simulink model "ELECTRIC_RC_AIRCRAFT_simulink_backup_3"  (R2025b)
settings: Solver=VariableStepAuto  StartTime=0.0  StopTime=1000  RelTol=1e-3
values from neighbouring files (symbols this model uses):
  AoA = [-5 0 5 10 15]    [ELECTRIC_RC_AIRCRAFT.m]
  C_mq = -2*((Tail_Wing_Area/Wing_Surface_Area)*(tail_moment_arm/chord_length_tail))    (= -0.900546448087)    [ELECTRIC_RC_AIRCRAFT.m]
  C_mse = -n*(Tail_Wing_Area/Wing_Surface_Area)*(tail_moment_arm/chord_length_tail)    (= -0.351213114754)    [ELECTRIC_RC_AIRCRAFT.m]
  chord_length = 0.25    [ELECTRIC_RC_AIRCRAFT.m]
  CL = [-0.249 0.205 0.752 1.190 1.316]    [ELECTRIC_RC_AIRCRAFT.m]
  CM = [0.0550 0.0260 -0.0854 -0.1805]    [ELECTRIC_RC_AIRCRAFT.m]
  g = 9.81    [ELECTRIC_RC_AIRCRAFT.m]
  Inertia = (m/12)*(fuselage_length^2+wing_span^2)    (= 0.54883225)    [ELECTRIC_RC_AIRCRAFT.m]
  m = 1.83    [ELECTRIC_RC_AIRCRAFT.m]
  Velocity_initial = 20    [ELECTRIC_RC_AIRCRAFT.m]
  Wing_Surface_Area = 0.4575    [ELECTRIC_RC_AIRCRAFT.m]
libraries: aerolibconvert2 x4, slpidlib x3, aerolibadyn x1, aerolibasang x1, aerolibbdyn x1, aerolibactuator x1, simulink x1, aerolibpropulsion2 x1
settings Model: Creator=papar  LastModifiedBy=papar

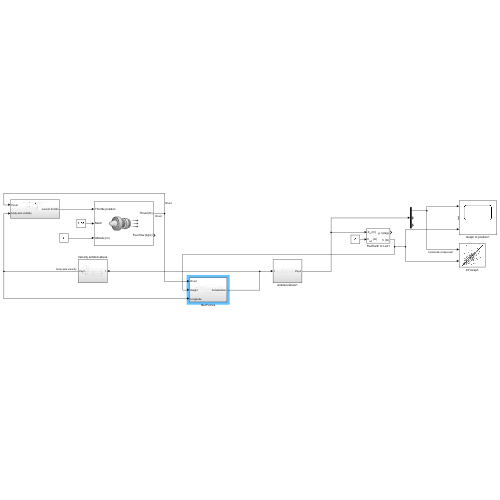
[thumbnail: Simulink's stored preview of the top-level diagram]
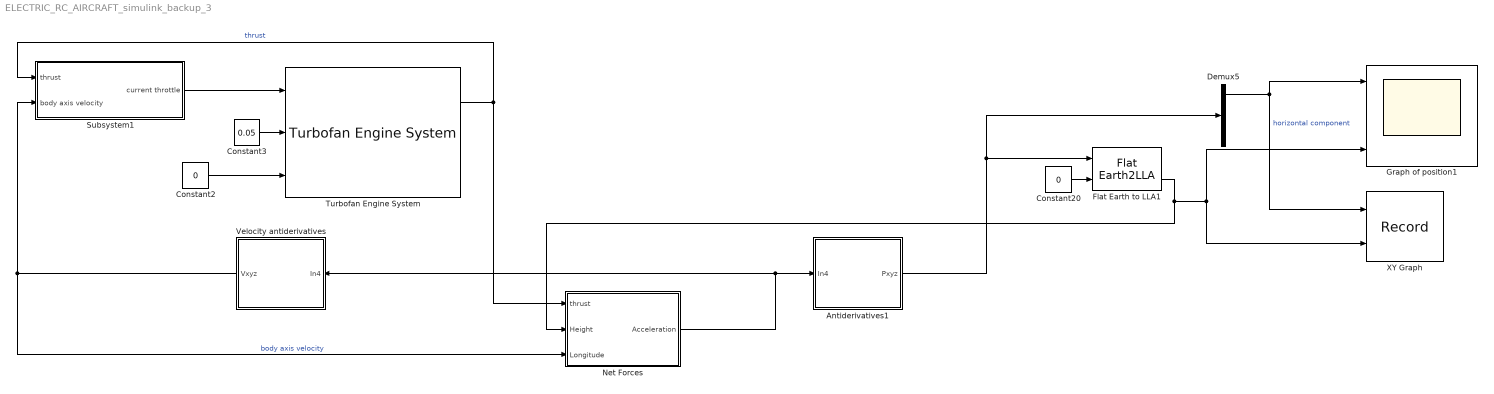
== system ELECTRIC_RC_AIRCRAFT_simulink_backup_3 ==
  Antiderivatives1 : Subsystem
  Constant2 : Constant  Value=0
  Constant20 : Constant  Value=0
  Constant3 : Constant  Value=0.05
  Demux5 : Demux  Outputs=3
  Flat Earth to LLA1 : FlatEarth2LLA
  Graph of position1 : Scope  NumInputPorts=3
      settings: ActiveDisplayYMinimum=-1.9016190813754986E+6  ActiveDisplayYMaximum=1.43321045610095E+6
  Net Forces : Subsystem
  Subsystem1 : Subsystem
  Turbofan Engine System : aerolibpropulsion2/Turbofan Engine System  units=Metric (MKS)  ic_source=Internal  IC=50  Fmax=50  tau=0.4  SFC=0  Nt=0.9
  Velocity antiderivatives : Subsystem
  XY Graph : Record  NumPorts=2.0  FileSettingsInternal="{\"entries\":[{\"content\":{\"excelSettings\":{\"content\":{},\"type\":\"Streamout.ExcelSettings\"},\"parquetSettings\":{\"content\":{},\"type\":\"Streamout.ParquetSettings\"}},\"type\":\"Streamout.FileSettingStorage\",\"uuid\":\"\"}],\"packageUris\":[\"http:\\/\\/schema.mathworks.com\\/mf0\\/streamout_blocks\\/R2020a\"],\"version\":\"1.0\"}"  FrameSettings=[0, 0]  Layout=[1 1]  SignalsInternal="{\"entries\":[{\"content\":{\"signals\":[{\"content\":{\"blockPath\":[],\"dimensions\":[1],\"domain\":\"\",\"lineColor\":\"#a2142f\",\"plots\":[ 1 ],\"port\":1,\"sid\":[\"\"],\"signalID\":1,\"signalName\":\"horizontal component\"},\"type\":\"RecordBlkView.Signal\",\"uuid\":\"\"},{\"content\":{\"blockPath\":[],\"dimensions\":[1],\"domain\":\"\",\"lineColor\":\"#139fff\",\"plots\":[ 1 ],\"port\":2,\"sid\":[\"\"],\"signalID\":2,\"signalName\":\"Flat Earth to LLA1:2\"},\"type\":\"RecordBlkView.Signal\",\"uuid\":\"\"}]},\"type\":\"RecordBlkView.InputSignals\",\"uuid\":\"\"}],\"packageUris\":[\"http:\\/\\/schema.mathworks.com\\/mf0\\/streamout_blocks\\/R2020a\"],\"version\":\"1.0\"}"  VisualizationBindings="{\"xyplotplugin\":{\"info\":[{\"series\":[{\"bindingParametersList\":[{\"parameter\":\"X-Axis\",\"signalID\":1,\"signalName\":\"horizontal component\"},{\"parameter\":\"Y-Axis\",\"signalID\":2,\"signalName\":\"Flat Earth to LLA1:2\"}],\"seriesID\":0}],\"subplotID\":1}]}}"  CompatibilityTag=XY
  wires:
  Constant2/1 -> Turbofan Engine System/3
  Constant3/1 -> Turbofan Engine System/2
  Antiderivatives1/1(Pxyz) -> Demux5/1, Flat Earth to LLA1/1
  Constant20/1 -> Flat Earth to LLA1/2
  Demux5/1 -> Graph of position1/1, XY Graph/1  "horizontal component"
  Flat Earth to LLA1/2 -> Net Forces/2(Height), Graph of position1/3, XY Graph/2
  Velocity antiderivatives/1(Vxyz) -> Net Forces/3(Longitude), Subsystem1/2(body axis velocity)  "body axis velocity"
  Net Forces/1(Acceleration) -> Antiderivatives1/1(In4), Velocity antiderivatives/1(In4)
  Turbofan Engine System/1 -> Subsystem1/1(thrust), Net Forces/1(thrust)  "thrust"
  Subsystem1/1(current throttle) -> Turbofan Engine System/1

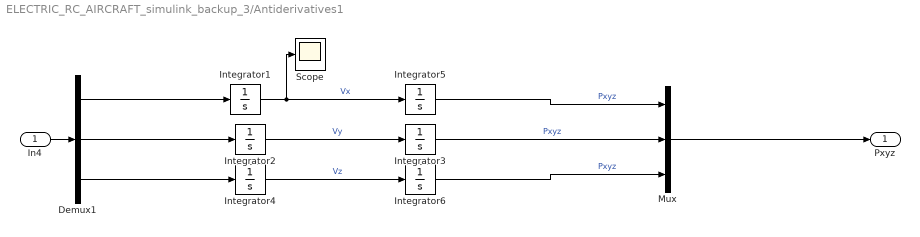
== system ELECTRIC_RC_AIRCRAFT_simulink_backup_3/Antiderivatives1 ==
  In4 : Inport
  Demux1 : Demux  Outputs=3
  Integrator1 : Integrator  InitialCondition=Velocity_initial  UpperSaturationLimit=30  LowerSaturationLimit=-10
  Integrator{2..6} (5 alike) : Integrator
  Mux : Mux  Inputs=3
  Scope : Scope
      settings: ActiveDisplayYMinimum=-71.95223956202382  ActiveDisplayYMaximum=46.668491481612783  DataLoggingVariableName=ScopeData4
  Pxyz : Outport
  wires:
  Integrator2/1 -> Integrator3/1  "Vy"
  In4/1 -> Demux1/1
  Integrator1/1 -> Scope/1, Integrator5/1  "Vx"
  Demux1/2 -> Integrator2/1
  Demux1/1 -> Integrator1/1
  Demux1/3 -> Integrator4/1
  Integrator4/1 -> Integrator6/1  "Vz"
  Mux/1 -> Pxyz/1
  Integrator3/1 -> Mux/2  "Pxyz"
  Integrator5/1 -> Mux/1  "Pxyz"
  Integrator6/1 -> Mux/3  "Pxyz"

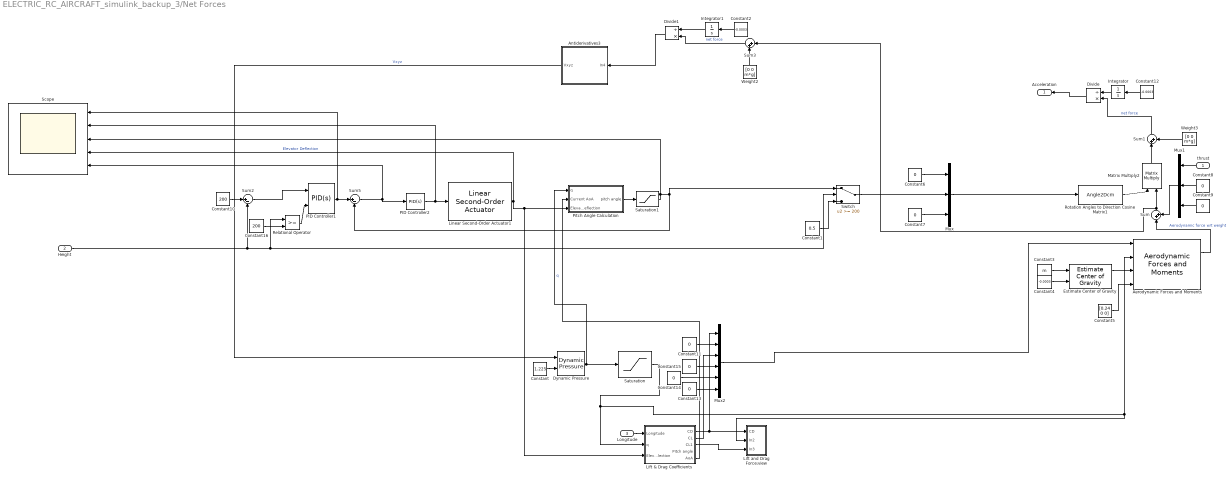
== system ELECTRIC_RC_AIRCRAFT_simulink_backup_3/Net Forces ==
  thrust : Inport
  Height : Inport  Port=2
  Longitude : Inport  Port=3
  "Aerodynamic Forces and Moments " : aerolibadyn/Aerodynamic Forces and Moments   inputAxes=Body  outputForceAxes=Body  outputMomentAxes=Body  S=Wing_Surface_Area  b=1.83  cbar=0.25
  Antiderivatives3 : Subsystem
  Constant : Constant  Value=1.225
  Constant1 : Constant  Value=0.5
  Constant10 : Constant  Value=200
  Constant{6..9,11,13..15} (8 alike) : Constant  Value=0
  Constant12 : Constant  Value=-0.0003
  Constant16 : Constant  Value=200
  Constant2 : Constant  Value=-0.0003
  Constant3 : Constant  Value=m
  Constant4 : Constant  Value=-0.0003
  Constant5 : Constant  Value=[0.24 0 0]
  Divide : Product  Inputs=/*
  Divide1 : Product  Inputs=/*
  Dynamic Pressure : aerolibasang/Dynamic Pressure
  Estimate Center of Gravity : aerolibbdyn/Estimate Center of Gravity  fmass=m  emass=1.63  fcg=[0.24 0 0]'  ecg=[0.23 0 0]'
  Integrator : Integrator  InitialCondition=m  LimitOutput=on  UpperSaturationLimit=1.83  LowerSaturationLimit=1.53
  Integrator1 : Integrator  InitialCondition=m  LimitOutput=on  UpperSaturationLimit=1.83  LowerSaturationLimit=1.53
  Lift & Drag Coefficients : Subsystem
  Lift and Drag Force:view : Subsystem
  Linear Second-Order Actuator1 : aerolibactuator/Linear Second-Order Actuator  wn_fin=8  z_fin=0.7  fin_act_0=0  fin_act_vel=0
  Matrix Multiply2 : Product  Multiplication=Matrix(*)
  Mux : Mux  Inputs=3
  Mux1 : Mux  Inputs=3
  Mux2 : Mux  Inputs=6
  PID Controller1 : slpidlib/PID Controller  Controller=PID  Form=Parallel  TimeDomain=Continuous-time  UseExternalTs=off  SampleTime=-1  IntegratorMethod=Forward Euler  FilterMethod=Forward Euler  ControllerParametersSource=internal  P=1.0E-2  I=0  UseKiTs=off  D=0  UseExternalDerivativeSource=off  N=10  UseFilter=on  TunerSelectOption=Transfer Function Based (PID Tuner App)  InitialConditionSource=internal  InitialConditionForIntegrator=0  InitialConditionForFilter=0  DifferentiatorICPrevScaledInput=0  ExternalReset=rising  TrackingMode=off  Kt=1  LimitOutput=on  SatLimitsSource=internal  UpperSaturationLimit=0.087  LowerSaturationLimit=-0.087  LinearizeAsGain=on  AntiWindupMode=none  Kb=1  LimitIntegrator=off  UpperIntegratorSaturationLimit=inf  LowerIntegratorSaturationLimit=-inf  POutMin=[]  POutMax=[]  IOutMin=[]  IOutMax=[]  DOutMin=[]  DOutMax=[]  NOutMin=[]  NOutMax=[]  SumOutMin=[]  SumOutMax=[]  SaturationOutMin=[]  SaturationOutMax=[]  PParamMin=[]  PParamMax=[]  IParamMin=[]  IParamMax=[]  DParamMin=[]  DParamMax=[]  NParamMin=[]  NParamMax=[]  KbParamMin=[]  KbParamMax=[]  KtParamMin=[]  KtParamMax=[]  KbOutMin=[]  KbOutMax=[]  KtOutMin=[]  KtOutMax=[]  IntegratorOutMin=[]  IntegratorOutMax=[]  FilterOutMin=[]  FilterOutMax=[]  SumI1OutMin=[]  SumI1OutMax=[]  SumI2OutMin=[]  SumI2OutMax=[]  SumI3OutMin=[]  SumI3OutMax=[]  SumI4OutMin=[]  SumI4OutMax=[]  SumDOutMin=[]  SumDOutMax=[]  DifferentiatorOutMin=[]  DifferentiatorOutMax=[]  FilterDiffOutCoefMin=[]  FilterDiffOutCoefMax=[]  ReciprocalOutMin=[]  ReciprocalOutMax=[]  SumDenOutMin=[]  SumDenOutMax=[]  SumNumOutMin=[]  SumNumOutMax=[]  DivideOutMin=[]  DivideOutMax=[]  UdiffTsProdOutMin=[]  UdiffTsProdOutMax=[]  NTsProdOutMin=[]  NTsProdOutMax=[]  UintegralTsProdOutMin=[]  UintegralTsProdOutMax=[]  UngainTsProdOutMin=[]  UngainTsProdOutMax=[]  ClampingZeroOutDataTypeStr=Inherit: Inherit via back propagation  ClampingZeroOutMin=[]  ClampingZeroOutMax=[]  FilterDenConstantOutDataTypeStr=Inherit: Inherit via back propagation  FilterDenConstantOutMin=[]  FilterDenConstantOutMax=[]  PCopyOutDataTypeStr=Inherit: Inherit via back propagation  PCopyOutMin=[]  PCopyOutMax=[]  NCopyOutDataTypeStr=Inherit: Inherit via back propagation  NCopyOutMin=[]  NCopyOutMax=[]  IntegratorContinuousStateAttributes=''  IntegratorStateMustResolveToSignalObject=off  IntegratorRTWStateStorageClass=Auto  FilterContinuousStateAttributes=''  FilterStateMustResolveToSignalObject=off  FilterRTWStateStorageClass=Auto  ParallelPVariant=InternalParameters  IdealPVariant=Disabled  IVariant=InternalParameters  DVariant=InternalParameters  IntegratorVariant=Continuous  SatVariant=Enabled  AWVariant=Passthrough  PCopyVariant=Disabled  TRVariant=Disabled  FdbkBlocksVariant=Forward  IdealPFdbkVariant=Disabled  SatFdbkVariant=Disabled  DerivativeFilterVariant=ContFilter  NVariant=InternalParameters  NCopyVariant=Disabled  FilterICVariant=InternalICsFilter  IntegratorICVariant=InternalICs  ExternalResetVariant=ExternalReset  TRSumVariant=Passthrough  SumFdbkVariant=Disabled  SumVariant=Sum_PID  TsampFilterVariant=InternalTs  TsampNgainVariant=Passthrough  TsampIntegralVariant=Disabled_SignalSpec  ExternalSaturationOutDataTypeStr=Inherit: Same as second input  DerivativeSourceVariant=ErrorSignal  PreIntVariant=InternalPreInt
  PID Controller2 : slpidlib/PID Controller  Controller=PID  Form=Parallel  TimeDomain=Continuous-time  UseExternalTs=off  SampleTime=-1  IntegratorMethod=Forward Euler  FilterMethod=Forward Euler  ControllerParametersSource=internal  P=1.0E-3  I=0  UseKiTs=off  D=1.0E-3  UseExternalDerivativeSource=off  N=20  UseFilter=on  TunerSelectOption=Transfer Function Based (PID Tuner App)  InitialConditionSource=internal  InitialConditionForIntegrator=0  InitialConditionForFilter=0  DifferentiatorICPrevScaledInput=0  ExternalReset=none  TrackingMode=off  Kt=1  LimitOutput=off  SatLimitsSource=internal  UpperSaturationLimit=inf  LowerSaturationLimit=-inf  LinearizeAsGain=on  AntiWindupMode=none  Kb=1  LimitIntegrator=off  UpperIntegratorSaturationLimit=inf  LowerIntegratorSaturationLimit=-inf  POutMin=[]  POutMax=[]  IOutMin=[]  IOutMax=[]  DOutMin=[]  DOutMax=[]  NOutMin=[]  NOutMax=[]  SumOutMin=[]  SumOutMax=[]  SaturationOutMin=[]  SaturationOutMax=[]  PParamMin=[]  PParamMax=[]  IParamMin=[]  IParamMax=[]  DParamMin=[]  DParamMax=[]  NParamMin=[]  NParamMax=[]  KbParamMin=[]  KbParamMax=[]  KtParamMin=[]  KtParamMax=[]  KbOutMin=[]  KbOutMax=[]  KtOutMin=[]  KtOutMax=[]  IntegratorOutMin=[]  IntegratorOutMax=[]  FilterOutMin=[]  FilterOutMax=[]  SumI1OutMin=[]  SumI1OutMax=[]  SumI2OutMin=[]  SumI2OutMax=[]  SumI3OutMin=[]  SumI3OutMax=[]  SumI4OutMin=[]  SumI4OutMax=[]  SumDOutMin=[]  SumDOutMax=[]  DifferentiatorOutMin=[]  DifferentiatorOutMax=[]  FilterDiffOutCoefMin=[]  FilterDiffOutCoefMax=[]  ReciprocalOutMin=[]  ReciprocalOutMax=[]  SumDenOutMin=[]  SumDenOutMax=[]  SumNumOutMin=[]  SumNumOutMax=[]  DivideOutMin=[]  DivideOutMax=[]  UdiffTsProdOutMin=[]  UdiffTsProdOutMax=[]  NTsProdOutMin=[]  NTsProdOutMax=[]  UintegralTsProdOutMin=[]  UintegralTsProdOutMax=[]  UngainTsProdOutMin=[]  UngainTsProdOutMax=[]  ClampingZeroOutDataTypeStr=Inherit: Inherit via back propagation  ClampingZeroOutMin=[]  ClampingZeroOutMax=[]  FilterDenConstantOutDataTypeStr=Inherit: Inherit via back propagation  FilterDenConstantOutMin=[]  FilterDenConstantOutMax=[]  PCopyOutDataTypeStr=Inherit: Inherit via back propagation  PCopyOutMin=[]  PCopyOutMax=[]  NCopyOutDataTypeStr=Inherit: Inherit via back propagation  NCopyOutMin=[]  NCopyOutMax=[]  IntegratorContinuousStateAttributes=''  IntegratorStateMustResolveToSignalObject=off  IntegratorRTWStateStorageClass=Auto  FilterContinuousStateAttributes=''  FilterStateMustResolveToSignalObject=off  FilterRTWStateStorageClass=Auto  ParallelPVariant=InternalParameters  IdealPVariant=Disabled  IVariant=InternalParameters  DVariant=InternalParameters  IntegratorVariant=Continuous  SatVariant=Disabled  AWVariant=Passthrough  PCopyVariant=Disabled  TRVariant=Disabled  FdbkBlocksVariant=Forward  IdealPFdbkVariant=Disabled  SatFdbkVariant=Disabled  DerivativeFilterVariant=ContFilter  NVariant=InternalParameters  NCopyVariant=Disabled  FilterICVariant=InternalICsFilter  IntegratorICVariant=InternalICs  ExternalResetVariant=Disabled  TRSumVariant=Passthrough  SumFdbkVariant=Disabled  SumVariant=Sum_PID  TsampFilterVariant=InternalTs  TsampNgainVariant=Passthrough  TsampIntegralVariant=Disabled_SignalSpec  ExternalSaturationOutDataTypeStr=Inherit: Same as second input  DerivativeSourceVariant=ErrorSignal  PreIntVariant=InternalPreInt
  Pitch Angle Calculation : Subsystem
  Relational Operator : RelationalOperator  OutDataTypeStr=boolean  RndMeth=Simplest  InputSameDT=off
  Rotation Angles to Direction Cosine Matrix1 : Angle2Dcm  rotationOrder=XYZ
      settings: AttributesFormatString=Rotation Order: %<rotationOrder>
  Saturation : Saturate  UpperLimit=200  LowerLimit=0
  Saturation1 : Saturate  UpperLimit=0.1  LowerLimit=-1.7
  Scope : Scope  NumInputPorts=5
      settings: ActiveDisplayYMinimum=-6.4413632870801404E+7  ActiveDisplayYMaximum=4.62135418449443E+7  DataLoggingVariableName=ScopeData2
  Sum : Sum  Inputs=|++
  Sum1 : Sum  Inputs=|++
  Sum2 : Sum  Inputs=|+-
  Sum3 : Sum  Inputs=|++
  Sum5 : Sum  Inputs=|+-
  Switch : Switch  Threshold=200  SaturateOnIntegerOverflow=off  InputSameDT=off
  Weight2 : Constant  Value=[0 0 m*g]
  Weight3 : Constant  Value=[0 0 m*g]
  Acceleration : Outport
  wires:
  Constant5/1 -> "Aerodynamic Forces and Moments "/4
  Saturation/1 -> Lift & Drag Coefficients/2(q), "Aerodynamic Forces and Moments "/2, Lift and Drag Force:view/2(In2)
  Lift & Drag Coefficients/1(CD) -> Mux2/1, Lift and Drag Force:view/1(CD)
  Longitude/1 -> Lift & Drag Coefficients/1(Longitude)
  Constant8/1 -> Mux1/2
  Constant/1 -> Dynamic Pressure/2
  Dynamic Pressure/1 -> Saturation/1, Pitch Angle Calculation/1(q)  "q"
  Rotation Angles to Direction Cosine Matrix1/1 -> Matrix Multiply2/1
  Mux1/1 -> Sum/2
  Constant10/1 -> Sum2/1
  Sum/1 -> Matrix Multiply2/2, Sum3/1
  Mux2/1 -> "Aerodynamic Forces and Moments "/1
  thrust/1 -> Mux1/1
  Constant11/1 -> Mux2/2
  Estimate Center of Gravity/1 -> "Aerodynamic Forces and Moments "/3
  Weight3/1 -> Sum1/2
  Constant14/1 -> Mux2/5
  Weight2/1 -> Sum3/2
  Antiderivatives3/1(Vxyz) -> Dynamic Pressure/1  "Vxyz"
  Constant6/1 -> Mux/1
  Lift & Drag Coefficients/3(CL1) -> Lift and Drag Force:view/3(In3)
  "Aerodynamic Forces and Moments "/1 -> Sum/1  "Aerodynamic force w/t weight"
  Constant7/1 -> Mux/3
  Matrix Multiply2/1 -> Sum1/1
  Constant9/1 -> Mux1/3
  Constant13/1 -> Mux2/6
  Constant15/1 -> Mux2/4
  Lift & Drag Coefficients/2(CL) -> Mux2/3
  Constant3/1 -> Estimate Center of Gravity/1
  Constant4/1 -> Estimate Center of Gravity/2
  Constant12/1 -> Integrator/1
  Integrator/1 -> Divide/1
  Divide/1 -> Acceleration/1
  Sum1/1 -> Divide/2  "net force"
  Sum3/1 -> Divide1/2  "net force"
  Integrator1/1 -> Divide1/1
  Constant2/1 -> Integrator1/1
  Divide1/1 -> Antiderivatives3/1(In4)
  PID Controller1/1 -> Scope/1, Sum5/1
  Sum5/1 -> PID Controller2/1, Scope/5
  Lift & Drag Coefficients/5(AoA) -> Pitch Angle Calculation/2(Current AoA)
  Pitch Angle Calculation/1(pitch angle) -> Saturation1/1
  Mux/1 -> Rotation Angles to Direction Cosine Matrix1/1
  PID Controller2/1 -> Scope/2, Linear Second-Order Actuator1/1
  Linear Second-Order Actuator1/1 -> Scope/4, Lift & Drag Coefficients/3(Elevator Deflection), Pitch Angle Calculation/3(Elevator Deflection)  "Elevator Deflection"
  Sum2/1 -> PID Controller1/1
  Switch/1 -> Mux/2
  Constant1/1 -> Switch/3
  Height/1 -> Relational Operator/1, Switch/2, Sum2/2
  Saturation1/1 -> Switch/1, Sum5/2, Scope/3
  Constant16/1 -> Relational Operator/2
  Relational Operator/1 -> PID Controller1/2

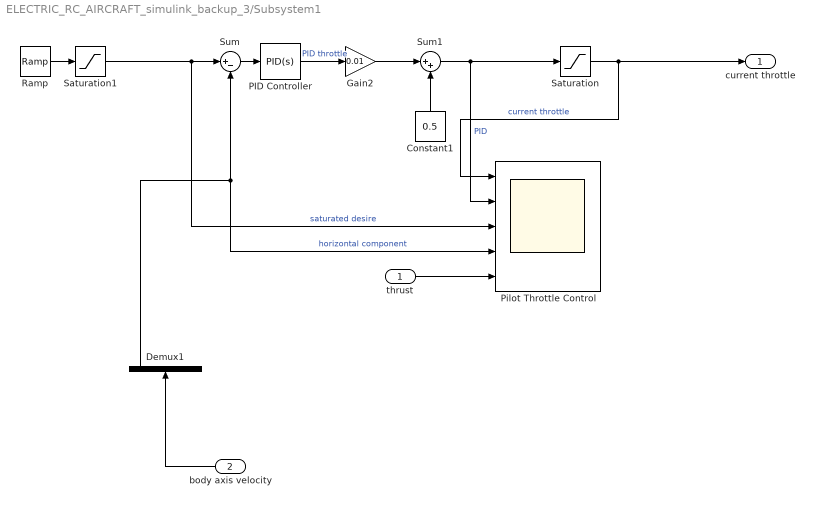
== system ELECTRIC_RC_AIRCRAFT_simulink_backup_3/Subsystem1 ==
  thrust : Inport
  body axis velocity : Inport  Port=2
  Constant1 : Constant  Value=0.5
  Demux1 : Demux  Outputs=3
  Gain2 : Gain  Gain=0.01
  PID Controller : slpidlib/PID Controller  Controller=PID  Form=Parallel  TimeDomain=Continuous-time  UseExternalTs=off  SampleTime=-1  IntegratorMethod=Forward Euler  FilterMethod=Forward Euler  ControllerParametersSource=internal  P=0.5  I=5.0E-3  UseKiTs=off  D=0.1  UseExternalDerivativeSource=off  N=20  UseFilter=on  TunerSelectOption=Transfer Function Based (PID Tuner App)  InitialConditionSource=internal  InitialConditionForIntegrator=0  InitialConditionForFilter=0  DifferentiatorICPrevScaledInput=0  ExternalReset=none  TrackingMode=off  Kt=1  LimitOutput=off  SatLimitsSource=internal  UpperSaturationLimit=inf  LowerSaturationLimit=-inf  LinearizeAsGain=on  AntiWindupMode=none  Kb=1  LimitIntegrator=off  UpperIntegratorSaturationLimit=inf  LowerIntegratorSaturationLimit=-inf  POutMin=[]  POutMax=[]  IOutMin=[]  IOutMax=[]  DOutMin=[]  DOutMax=[]  NOutMin=[]  NOutMax=[]  SumOutMin=[]  SumOutMax=[]  SaturationOutMin=[]  SaturationOutMax=[]  PParamMin=[]  PParamMax=[]  IParamMin=[]  IParamMax=[]  DParamMin=[]  DParamMax=[]  NParamMin=[]  NParamMax=[]  KbParamMin=[]  KbParamMax=[]  KtParamMin=[]  KtParamMax=[]  KbOutMin=[]  KbOutMax=[]  KtOutMin=[]  KtOutMax=[]  IntegratorOutMin=[]  IntegratorOutMax=[]  FilterOutMin=[]  FilterOutMax=[]  SumI1OutMin=[]  SumI1OutMax=[]  SumI2OutMin=[]  SumI2OutMax=[]  SumI3OutMin=[]  SumI3OutMax=[]  SumI4OutMin=[]  SumI4OutMax=[]  SumDOutMin=[]  SumDOutMax=[]  DifferentiatorOutMin=[]  DifferentiatorOutMax=[]  FilterDiffOutCoefMin=[]  FilterDiffOutCoefMax=[]  ReciprocalOutMin=[]  ReciprocalOutMax=[]  SumDenOutMin=[]  SumDenOutMax=[]  SumNumOutMin=[]  SumNumOutMax=[]  DivideOutMin=[]  DivideOutMax=[]  UdiffTsProdOutMin=[]  UdiffTsProdOutMax=[]  NTsProdOutMin=[]  NTsProdOutMax=[]  UintegralTsProdOutMin=[]  UintegralTsProdOutMax=[]  UngainTsProdOutMin=[]  UngainTsProdOutMax=[]  ClampingZeroOutDataTypeStr=Inherit: Inherit via back propagation  ClampingZeroOutMin=[]  ClampingZeroOutMax=[]  FilterDenConstantOutDataTypeStr=Inherit: Inherit via back propagation  FilterDenConstantOutMin=[]  FilterDenConstantOutMax=[]  PCopyOutDataTypeStr=Inherit: Inherit via back propagation  PCopyOutMin=[]  PCopyOutMax=[]  NCopyOutDataTypeStr=Inherit: Inherit via back propagation  NCopyOutMin=[]  NCopyOutMax=[]  IntegratorContinuousStateAttributes=''  IntegratorStateMustResolveToSignalObject=off  IntegratorRTWStateStorageClass=Auto  FilterContinuousStateAttributes=''  FilterStateMustResolveToSignalObject=off  FilterRTWStateStorageClass=Auto  ParallelPVariant=InternalParameters  IdealPVariant=Disabled  IVariant=InternalParameters  DVariant=InternalParameters  IntegratorVariant=Continuous  SatVariant=Disabled  AWVariant=Passthrough  PCopyVariant=Disabled  TRVariant=Disabled  FdbkBlocksVariant=Forward  IdealPFdbkVariant=Disabled  SatFdbkVariant=Disabled  DerivativeFilterVariant=ContFilter  NVariant=InternalParameters  NCopyVariant=Disabled  FilterICVariant=InternalICsFilter  IntegratorICVariant=InternalICs  ExternalResetVariant=Disabled  TRSumVariant=Passthrough  SumFdbkVariant=Disabled  SumVariant=Sum_PID  TsampFilterVariant=InternalTs  TsampNgainVariant=Passthrough  TsampIntegralVariant=Disabled_SignalSpec  ExternalSaturationOutDataTypeStr=Inherit: Same as second input  DerivativeSourceVariant=ErrorSignal  PreIntVariant=InternalPreInt
  Pilot Throttle Control : Scope  NumInputPorts=5
      settings: ActiveDisplayYMinimum=-82.386401039408824  ActiveDisplayYMaximum=23.931783016510508  DataLoggingVariableName=ScopeData2
  Ramp : simulink/Sources/Ramp  slope=-0.3  start=0  InitialOutput=700
  Saturation : Saturate  UpperLimit=1  LowerLimit=0
  Saturation1 : Saturate  UpperLimit=700  LowerLimit=500
  Sum : Sum  Inputs=|+-
  Sum1 : Sum  Inputs=|++
  current throttle : Outport
  wires:
  Ramp/1 -> Saturation1/1
  Sum1/1 -> Pilot Throttle Control/2, Saturation/1  "PID"
  Constant1/1 -> Sum1/2
  Gain2/1 -> Sum1/1
  Demux1/1 -> Pilot Throttle Control/4, Sum/2  "horizontal component"
  Saturation1/1 -> Pilot Throttle Control/3, Sum/1  "saturated desire"
  Saturation/1 -> Pilot Throttle Control/1, current throttle/1  "current throttle"
  PID Controller/1 -> Gain2/1  "PID throttle"
  Sum/1 -> PID Controller/1
  body axis velocity/1 -> Demux1/1
  thrust/1 -> Pilot Throttle Control/5

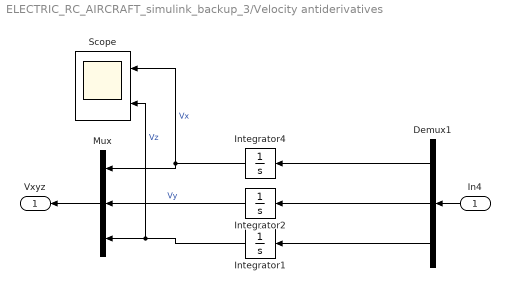
== system ELECTRIC_RC_AIRCRAFT_simulink_backup_3/Velocity antiderivatives ==
  In4 : Inport
  Demux1 : Demux  Outputs=3
  Integrator1 : Integrator
  Integrator2 : Integrator
  Integrator4 : Integrator  InitialCondition=Velocity_initial  UpperSaturationLimit=30  LowerSaturationLimit=-10
  Mux : Mux  Inputs=3
  Scope : Scope  NumInputPorts=2
      settings: ActiveDisplayYMinimum=-922.98167700183922  ActiveDisplayYMaximum=3421.7708124530582  DataLoggingVariableName=ScopeData3
  Vxyz : Outport
  wires:
  Mux/1 -> Vxyz/1
  Integrator4/1 -> Scope/1, Mux/1  "Vx"
  Demux1/3 -> Integrator1/1
  Demux1/1 -> Integrator4/1
  Demux1/2 -> Integrator2/1
  Integrator1/1 -> Scope/2, Mux/3  "Vz"
  In4/1 -> Demux1/1
  Integrator2/1 -> Mux/2  "Vy"

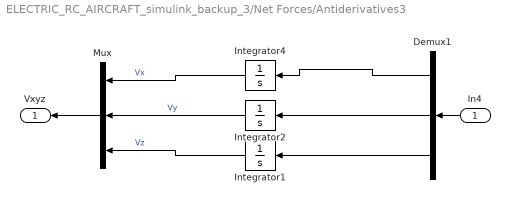
== system ELECTRIC_RC_AIRCRAFT_simulink_backup_3/Net Forces/Antiderivatives3 ==
  In4 : Inport
  Demux1 : Demux  Outputs=3
  Integrator1 : Integrator
  Integrator2 : Integrator
  Integrator4 : Integrator  InitialCondition=Velocity_initial  UpperSaturationLimit=30  LowerSaturationLimit=-10
  Mux : Mux  Inputs=3
  Vxyz : Outport
  wires:
  Integrator2/1 -> Mux/2  "Vy"
  In4/1 -> Demux1/1
  Integrator1/1 -> Mux/3  "Vz"
  Demux1/2 -> Integrator2/1
  Demux1/1 -> Integrator4/1
  Demux1/3 -> Integrator1/1
  Integrator4/1 -> Mux/1  "Vx"
  Mux/1 -> Vxyz/1

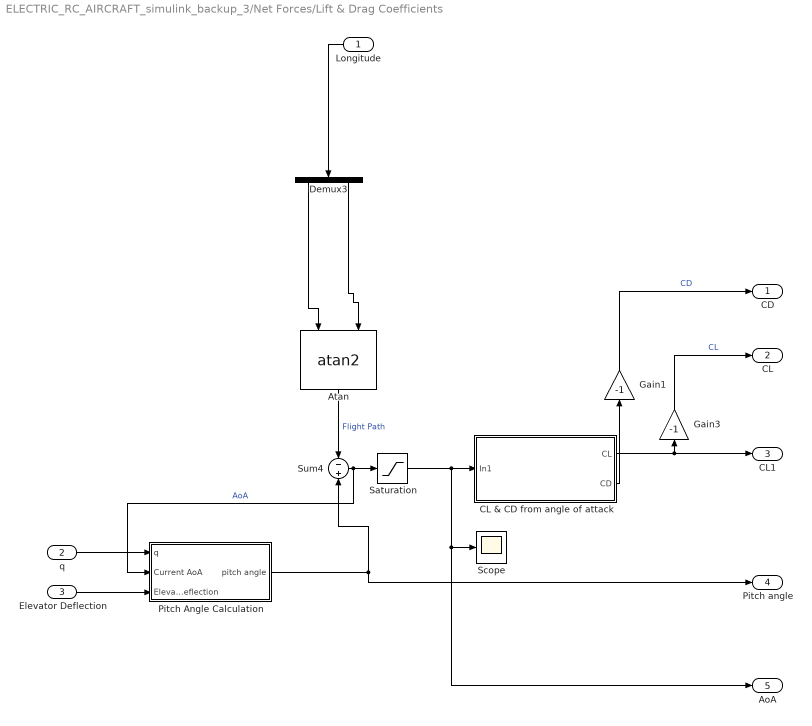
== system ELECTRIC_RC_AIRCRAFT_simulink_backup_3/Net Forces/Lift & Drag Coefficients ==
  Longitude : Inport
  q : Inport  Port=2
  Elevator Deflection : Inport  Port=3
  Atan : Trigonometry  Operator=atan2
  CL & CD from angle of attack : Subsystem
  Demux3 : Demux  Outputs=3
  Gain1 : Gain  Gain=-1
  Gain3 : Gain  Gain=-1
  Pitch Angle Calculation : Subsystem
  Saturation : Saturate  UpperLimit=2  LowerLimit=-2
  Scope : Scope
      settings: ActiveDisplayYMinimum=-7.4396684290622461E+11  ActiveDisplayYMaximum=1.1524832318855518E+12  DataLoggingVariableName=ScopeData6
  Sum4 : Sum  Inputs=-+
  CD : Outport
  CL : Outport  Port=2
  CL1 : Outport  Port=3
  Pitch angle : Outport  Port=4
  AoA : Outport  Port=5
  wires:
  Gain3/1 -> CL/1  "CL"
  Demux3/3 -> Atan/2
  Pitch Angle Calculation/1(pitch angle) -> Pitch angle/1, Sum4/2
  CL & CD from angle of attack/1(CL) -> CL1/1, Gain3/1
  Atan/1 -> Sum4/1  "Flight Path"
  Demux3/1 -> Atan/1
  Sum4/1 -> Pitch Angle Calculation/2(Current AoA), Saturation/1  "AoA"
  CL & CD from angle of attack/2(CD) -> Gain1/1
  q/1 -> Pitch Angle Calculation/1(q)
  Gain1/1 -> CD/1  "CD"
  Longitude/1 -> Demux3/1
  Saturation/1 -> Scope/1, AoA/1, CL & CD from angle of attack/1(In1)
  Elevator Deflection/1 -> Pitch Angle Calculation/3(Elevator Deflection)

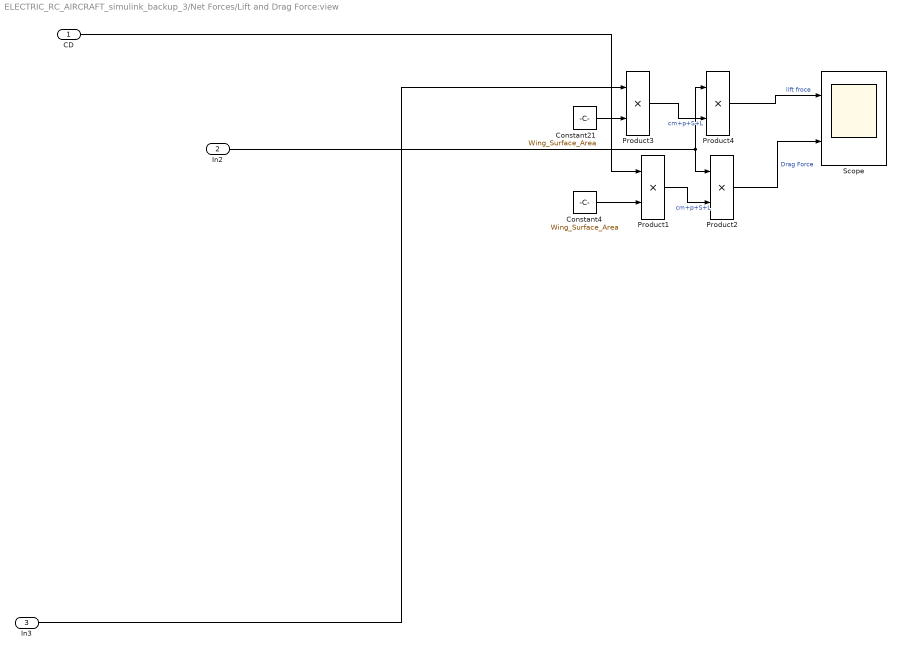
== system ELECTRIC_RC_AIRCRAFT_simulink_backup_3/Net Forces/Lift and Drag Force:view ==
  CD : Inport
  In2 : Inport  Port=2
  In3 : Inport  Port=3
  Constant21 : Constant  Value=Wing_Surface_Area
  Constant4 : Constant  Value=Wing_Surface_Area
  Product{1..4} (4 alike) : Product
  Scope : Scope  NumInputPorts=2
      settings: ActiveDisplayYMinimum=-12.927989400090087  ActiveDisplayYMaximum=37.993869481760044
  wires:
  Constant4/1 -> Product1/2
  Product2/1 -> Scope/2  "Drag Force"
  Product1/1 -> Product2/2  "cm+p+S+L"
  In2/1 -> Product4/1, Product2/1
  CD/1 -> Product1/1
  Constant21/1 -> Product3/2
  Product3/1 -> Product4/2  "cm+p+S+L"
  In3/1 -> Product3/1
  Product4/1 -> Scope/1  "lift froce"

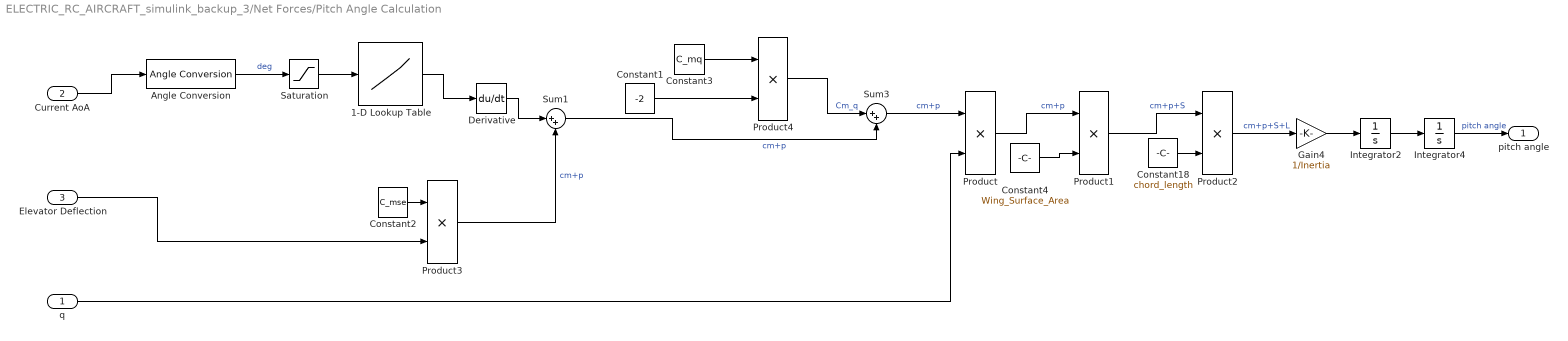
== system ELECTRIC_RC_AIRCRAFT_simulink_backup_3/Net Forces/Pitch Angle Calculation ==
  q : Inport
  Current AoA : Inport  Port=2
  Elevator Deflection : Inport  Port=3
  1-D Lookup Table : Lookup_n-D  NumberOfTableDimensions=1  BreakpointsForDimension1=[-5 0 5 10]  Table=CM  InternalRulePriority=Speed  RndMeth=Simplest
  Angle Conversion : aerolibconvert2/Angle Conversion  IU=rad  OU=deg
  Constant1 : Constant  Value=-2
  Constant18 : Constant  Value=chord_length
  Constant2 : Constant  Value=C_mse
  Constant3 : Constant  Value=C_mq
  Constant4 : Constant  Value=Wing_Surface_Area
  Derivative : Derivative
  Gain4 : Gain  Gain=1/Inertia
  Integrator2 : Integrator
  Integrator4 : Integrator
  Product{,1..4} (5 alike) : Product
  Saturation : Saturate  UpperLimit=10  LowerLimit=-10
  Sum1 : Sum  Inputs=|++
  Sum3 : Sum  Inputs=|++
  pitch angle : Outport
  wires:
  Product/1 -> Product1/1  "cm+p"
  Constant18/1 -> Product2/2
  Product1/1 -> Product2/1  "cm+p+S"
  Current AoA/1 -> Angle Conversion/1
  Constant4/1 -> Product1/2
  Integrator2/1 -> Integrator4/1
  Gain4/1 -> Integrator2/1
  q/1 -> Product/2
  Integrator4/1 -> pitch angle/1  "pitch angle"
  Saturation/1 -> 1-D Lookup Table/1
  Product2/1 -> Gain4/1  "cm+p+S+L"
  Angle Conversion/1 -> Saturation/1  "deg"
  1-D Lookup Table/1 -> Derivative/1
  Derivative/1 -> Sum1/1
  Sum1/1 -> Sum3/2  "cm+p"
  Elevator Deflection/1 -> Product3/2
  Constant1/1 -> Product4/2
  Product4/1 -> Sum3/1  "Cm_q"
  Constant2/1 -> Product3/1
  Product3/1 -> Sum1/2  "cm+p"
  Constant3/1 -> Product4/1
  Sum3/1 -> Product/1  "cm+p"

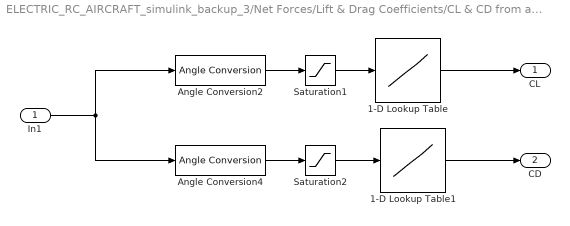
== system ELECTRIC_RC_AIRCRAFT_simulink_backup_3/Net Forces/Lift & Drag Coefficients/CL & CD from angle of attack ==
  In1 : Inport
  1-D Lookup Table : Lookup_n-D  NumberOfTableDimensions=1  BreakpointsForDimension1=AoA  Table=CL  InternalRulePriority=Speed  RndMeth=Simplest
  1-D Lookup Table1 : Lookup_n-D  NumberOfTableDimensions=1  BreakpointsForDimension1=AoA  Table=CL  InternalRulePriority=Speed  RndMeth=Simplest
  Angle Conversion2 : aerolibconvert2/Angle Conversion  IU=rad  OU=deg
  Angle Conversion4 : aerolibconvert2/Angle Conversion  IU=rad  OU=deg
  Saturation1 : Saturate  UpperLimit=0.15  LowerLimit=-0.05
  Saturation2 : Saturate  UpperLimit=0.15  LowerLimit=-0.05
  CL : Outport
  CD : Outport  Port=2
  wires:
  Angle Conversion2/1 -> Saturation1/1
  Angle Conversion4/1 -> Saturation2/1
  1-D Lookup Table1/1 -> CD/1
  1-D Lookup Table/1 -> CL/1
  In1/1 -> Angle Conversion4/1, Angle Conversion2/1
  Saturation1/1 -> 1-D Lookup Table/1
  Saturation2/1 -> 1-D Lookup Table1/1

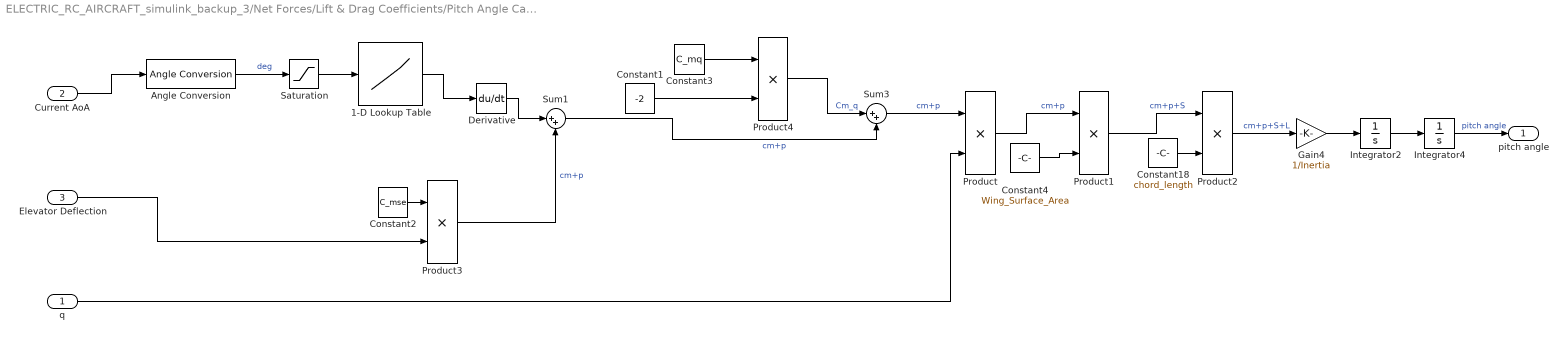
== system ELECTRIC_RC_AIRCRAFT_simulink_backup_3/Net Forces/Lift & Drag Coefficients/Pitch Angle Calculation ==
  q : Inport
  Current AoA : Inport  Port=2
  Elevator Deflection : Inport  Port=3
  1-D Lookup Table : Lookup_n-D  NumberOfTableDimensions=1  BreakpointsForDimension1=[-5 0 5 10]  Table=CM  InternalRulePriority=Speed  RndMeth=Simplest
  Angle Conversion : aerolibconvert2/Angle Conversion  IU=rad  OU=deg
  Constant1 : Constant  Value=-2
  Constant18 : Constant  Value=chord_length
  Constant2 : Constant  Value=C_mse
  Constant3 : Constant  Value=C_mq
  Constant4 : Constant  Value=Wing_Surface_Area
  Derivative : Derivative
  Gain4 : Gain  Gain=1/Inertia
  Integrator2 : Integrator
  Integrator4 : Integrator
  Product{,1..4} (5 alike) : Product
  Saturation : Saturate  UpperLimit=10  LowerLimit=-10
  Sum1 : Sum  Inputs=|++
  Sum3 : Sum  Inputs=|++
  pitch angle : Outport
  wires:
  Product/1 -> Product1/1  "cm+p"
  Constant18/1 -> Product2/2
  Product1/1 -> Product2/1  "cm+p+S"
  Current AoA/1 -> Angle Conversion/1
  Constant4/1 -> Product1/2
  Integrator2/1 -> Integrator4/1
  Gain4/1 -> Integrator2/1
  q/1 -> Product/2
  Integrator4/1 -> pitch angle/1  "pitch angle"
  Saturation/1 -> 1-D Lookup Table/1
  Product2/1 -> Gain4/1  "cm+p+S+L"
  Angle Conversion/1 -> Saturation/1  "deg"
  1-D Lookup Table/1 -> Derivative/1
  Derivative/1 -> Sum1/1
  Sum1/1 -> Sum3/2  "cm+p"
  Elevator Deflection/1 -> Product3/2
  Constant1/1 -> Product4/2
  Product4/1 -> Sum3/1  "Cm_q"
  Constant2/1 -> Product3/1
  Product3/1 -> Sum1/2  "cm+p"
  Constant3/1 -> Product4/1
  Sum3/1 -> Product/1  "cm+p"
